simulink model "reference_tracking"  (R2015a)
settings: Solver=ode45  StartTime=0.0  StopTime=20  RelTol=1e-3
values from neighbouring files (symbols this model uses):
  a = b0*(natural_freq(i)^2)    [autotuning_script.m]    (also in autotuning_v2.m)
  b = 2*natural_freq(i)*damping_ratio(j)    [autotuning_script.m]    (also in autotuning_v2.m)
  c = natural_freq(i)^2    [autotuning_script.m]    (also in autotuning_v2.m)
  ki = (rand+0.2)*ki    [autotuning_script.m]    (also in autotuning_v2.m = gains(index(1),2))
  kp = (rand+0.2)*kp    [autotuning_script.m]    (also in autotuning_v2.m = gains(index(1),1))
libraries: simulink x1
settings Model: Creator=dimtsoun  LastModifiedBy=dimtsoun

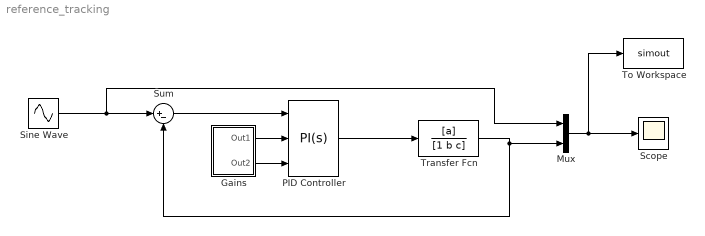
== system reference_tracking ==
  Gains : Subsystem
  Mux : Mux  Inputs=2
  PID Controller : simulink/Continuous/PID Controller  Controller=PI  TimeDomain=Continuous-time  SampleTime=-1  IntegratorMethod=Forward Euler  FilterMethod=Forward Euler  Form=Parallel  UseFilter=on  ControllerParametersSource=external  P=1  I=1  D=0  N=100  InitialConditionSource=internal  InitialConditionForIntegrator=0  InitialConditionForFilter=0  ExternalReset=none  LimitOutput=off  UpperSaturationLimit=inf  LowerSaturationLimit=-inf  LinearizeAsGain=on  AntiWindupMode=none  Kb=1  TrackingMode=off  Kt=1  PParamMin=[]  PParamMax=[]  IParamMin=[]  IParamMax=[]  DParamMin=[]  DParamMax=[]  NParamMin=[]  NParamMax=[]  KbParamMin=[]  KbParamMax=[]  KtParamMin=[]  KtParamMax=[]  POutMin=[]  POutMax=[]  IOutMin=[]  IOutMax=[]  DOutMin=[]  DOutMax=[]  NOutMin=[]  NOutMax=[]  KbOutMin=[]  KbOutMax=[]  KtOutMin=[]  KtOutMax=[]  IntegratorOutMin=[]  IntegratorOutMax=[]  FilterOutMin=[]  FilterOutMax=[]  SumOutMin=[]  SumOutMax=[]  SumI1OutMin=[]  SumI1OutMax=[]  SumI2OutMin=[]  SumI2OutMax=[]  SumI3OutMin=[]  SumI3OutMax=[]  SumDOutMin=[]  SumDOutMax=[]  SaturationOutMin=[]  SaturationOutMax=[]  IntegratorContinuousStateAttributes=''  IntegratorStateMustResolveToSignalObject=off  IntegratorRTWStateStorageClass=Auto  FilterContinuousStateAttributes=''  FilterStateMustResolveToSignalObject=off  FilterRTWStateStorageClass=Auto  DifferentiatorICPrevScaledInput=0  DifferentiatorOutMin=[]  DifferentiatorOutMax=[]
  Scope : Scope
  Sine Wave : Sin  SampleTime=0
  Sum : Sum  Inputs=|+-
  To Workspace : ToWorkspace  VariableName=simout  SaveFormat=Structure With Time  SampleTime=-1
  Transfer Fcn : TransferFcn  Numerator=[a]  Denominator=[1 b c]
  wires:
  Sine Wave/1 -> Mux/1, Sum/1
  Sum/1 -> PID Controller/1
  Gains/1(Out1) -> PID Controller/2
  Gains/2(Out2) -> PID Controller/3
  PID Controller/1 -> Transfer Fcn/1
  Transfer Fcn/1 -> Mux/2, Sum/2
  Mux/1 -> To Workspace/1, Scope/1

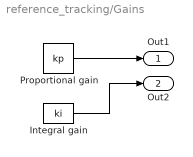
== system reference_tracking/Gains ==
  Integral gain : Constant  Value=ki
  Proportional gain : Constant  Value=kp
  Out1 : Outport
  Out2 : Outport  Port=2
  wires:
  Integral gain/1 -> Out2/1
  Proportional gain/1 -> Out1/1
